simulink model "pv_model"  (R2020a)
settings: Solver=VariableStepAuto  StartTime=0.0  StopTime=10  RelTol=1e-3
undefined symbols (not defined in the file): Eg0, Isc, K, Ki, n, Ns, q, Rs, Rsh, sigbuilder_block, Tn, Voc
libraries: powerlib x12, simulink x11, re_lib x1
settings Model: Creator=vardh  LastModifiedBy=sameeraa
settings SolverCC: AlgebraicLoopSolver=LineSearch
settings DebuggingCC: AlgebraicLoopMsg=none

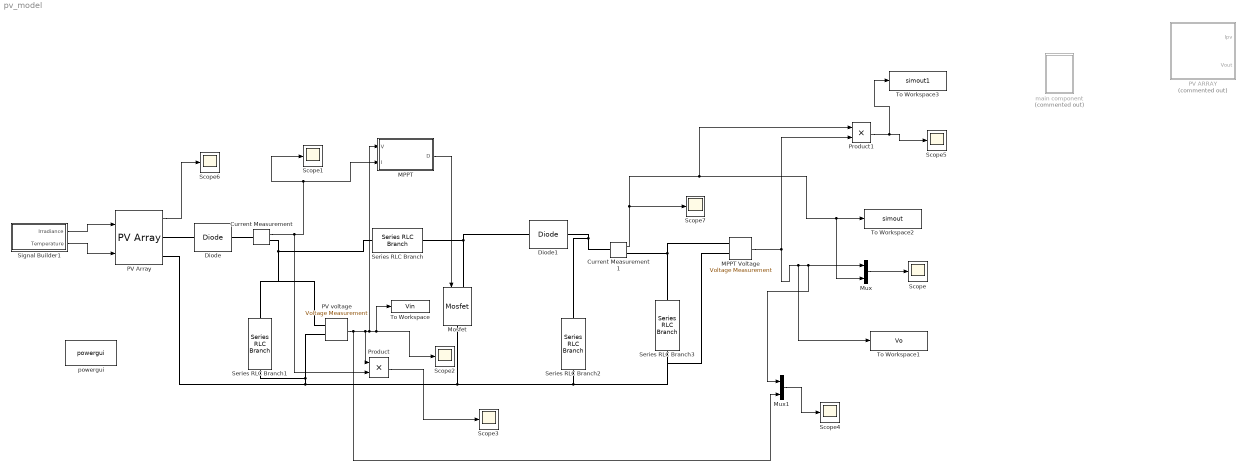
== system pv_model ==
  Current Measurement : powerlib/Measurements/Current Measurement  PhasorSimulation=off  OutputType=Complex  PSBequivalent=0
  Current Measurement1 : powerlib/Measurements/Current Measurement  PhasorSimulation=off  OutputType=Complex  PSBequivalent=0
  Diode : powerlib/Power Electronics/Diode  Ron=0.001  Lon=0  Vf=0.8  IC=0  UseSnubber=0  Rs=500  Cs=250e-9  Measurements=off
  Diode1 : powerlib/Power Electronics/Diode  Ron=0.001  Lon=0  Vf=0.8  IC=0  UseSnubber=0  Rs=500  Cs=250e-9  Measurements=off
  MPPT : Subsystem
  MPPT Voltage : powerlib/Measurements/Voltage Measurement  PhasorSimulation=off  OutputType=Complex  PSBequivalent=0
  Mosfet : powerlib/Power Electronics/Mosfet  Ron=0.1  Lon=0  Rd=0.01  Vfd=0  IC=0  Rs=1e5  Cs=inf  Measurements=off
  Mux : Mux  Inputs=2
  Mux1 : Mux  Inputs=2
  PV ARRAY : Subsystem  Commented=on
  PV Array : re_lib/Solar/PV Array  Npar=1  Nser=1  PlotType=one module @ 25 deg.C & specified irradiances  S_vec="[ 1000  800  600 ]"  Temp_C_vec="[ 45 25  ]"  ModuleName=User-defined  PlotWhenSelected=off  Pm=223.3  Ncell=60  Voc=36.3  Isc=7.84  Vm=29  Im=7.7  beta_Voc_pc=-0.36099  alpha_Isc_pc=0.102  beta_Voc=-0.13104  alpha_Isc=0.0079968  IL=8.0515  I0=2.9406e-10  nI=0.97985  Rsh=6175.6519  Rs=0.38059  RobustModel=off  RobustCellTemperature=25  BAL=on  Tc=1e-6  Tfilter=5e-5
  PV voltage : powerlib/Measurements/Voltage Measurement  PhasorSimulation=off  OutputType=Complex  PSBequivalent=0
  Product : Product
  Product1 : Product
  Scope{,1..7} (8 alike) : Scope
  Series RLC Branch : powerlib/Elements/Series RLC Branch  LConnTagsString=__new0  RConnTagsString=__new0  BranchType=L  Resistance=1  Inductance=1e-3  SetiL0=off  InitialCurrent=0  Capacitance=1e-6  Setx0=off  InitialVoltage=0  Measurements=None
  Series RLC Branch1 : powerlib/Elements/Series RLC Branch  LConnTagsString=__new0  RConnTagsString=__new0  BranchType=C  Resistance=1  Inductance=1e-3  SetiL0=off  InitialCurrent=0  Capacitance=1e-6  Setx0=off  InitialVoltage=0  Measurements=None
  Series RLC Branch2 : powerlib/Elements/Series RLC Branch  LConnTagsString=__new0  RConnTagsString=__new0  BranchType=C  Resistance=1  Inductance=1e-3  SetiL0=off  InitialCurrent=0  Capacitance=1e-6  Setx0=off  InitialVoltage=0  Measurements=None
  Series RLC Branch3 : powerlib/Elements/Series RLC Branch  LConnTagsString=__new0  RConnTagsString=__new0  BranchType=R  Resistance=1  Inductance=1e-3  SetiL0=off  InitialCurrent=0  Capacitance=1e-6  Setx0=off  InitialVoltage=0  Measurements=None
  Signal Builder1 : Subsystem  Tag=STV Subsys  LoadFcn=sigbuilder_block('load');  StartFcn=sigbuilder_block('start');  StopFcn=sigbuilder_block('stop');  ClipboardFcn=sigbuilder_block('clipboard');  mask(Sigbuilder block){tuvar=[0:10]}
      mask help: Simulink:masks:SigbuilderBlock_MD
      mask init:
      | if ~strcmp(get_param(bdroot(gcbh),'SimulationStatus'),'stopped') tuvar = sigbuilder_block('maskInit'); end
      settings: CopyFcn=sigbuilder_block('copy');  DeleteFcn=sigbuilder_block('delete');  ModelCloseFcn=sigbuilder_block('modelClose');  PreSaveFcn=sigbuilder_block('preSave');  PauseFcn=sigbuilder_block('pause');  ContinueFcn=sigbuilder_block('continue');  NameChangeFcn=sigbuilder_block('namechange');  OpenFcn=sigbuilder_block('open',[382.8 123 550.8 400.2 ]);  CloseFcn=sigbuilder_block('close');
      mask Display: plot(0, 0, 100, 100,[2, 2, 32, 32, 2], [68, 8, 8, 68, 68],[32, 2], [38, 38], [32, 19, 2],[53, 60, 44], [32, 17, 17, 2],[16, 16, 31, 31]);txt = getActiveGroup(gcbh);text(2, 100, txt,'verticalAlignment', 'top');
  To Workspace : ToWorkspace  VariableName=Vin  SampleTime=-1
  To Workspace1 : ToWorkspace  VariableName=Vo  SampleTime=-1
  To Workspace2 : ToWorkspace  VariableName=simout  SaveFormat=Timeseries  SampleTime=-1
  To Workspace3 : ToWorkspace  VariableName=simout1  SaveFormat=Timeseries  SampleTime=-1
  main component : Subsystem  Commented=on
  powergui : powerlib/powergui  Priority=1  SimulationMode=Continuous  SampleTime=50e-6  frequency=60  Iterations=50  frequencyindice=0  Pbase=100e6  ErrMax=1e-4  UnitsV=kV  UnitsW=MW  buscounter=0  FunctionMessages=off  echomessages=off  EnableUseOfTLC=off  CurrentSourceSwitches=off  DisableSnubberDevices=off  DisableRonSwitches=off  DisableVfSwitches=off  DisplayEquations=off  AutomaticDiscreteSolvers=off  SolverType=Tustin/Backward Euler (TBE)  Interpol=off  ExternalGateDelay=off  methode=off  Ts=100  x0status=blocks  SPID=on  SwTol=0  HookPort=off  NonlinearTolerance=1e-4  nMaxIteration=100  ContinueOnMaxIteration=off  RestoreLinks=warning  ResistiveCurrentMeasurement=off  Frange=[0:2:500]  Ylog=off  Xlog=on  ShowGrid=off  save=off  variable=ZData  structure=0  ZoomFFT=off  StartTime=0.0  cycles=1  DisplayStyle=1  fundamental=60  FreqAxis=off  MaxFrequency=1000  frequencyindicesteady=1  RmsSteady=1  display=off
  wires:
  Signal Builder1/1(Irradiance) -> PV Array/1
  Signal Builder1/2(Temperature) -> PV Array/2
  Current Measurement/1 -> Product/2, Scope1/1, MPPT/2(I)
  MPPT/1(D) -> Mosfet/1
  PV voltage/1 -> Scope2/1, To Workspace/1, MPPT/1(V), Product/1, Mux1/2
  Product/1 -> Scope3/1
  MPPT Voltage/1 -> To Workspace1/1, Mux/1, Mux1/1, Product1/2
  Mux/1 -> Scope/1
  Mux1/1 -> Scope4/1
  Current Measurement1/1 -> Scope7/1, Product1/1, To Workspace2/1, Mux/2
  Product1/1 -> To Workspace3/1, Scope5/1
  PV Array/1 -> Scope6/1
  connections:
  Diode/RConn1 -- Current Measurement/LConn1
  PV Array/RConn1 -- Diode/LConn1
  Series RLC Branch/LConn1 -- Current Measurement/RConn1 -- PV voltage/LConn1 -- Series RLC Branch1/LConn1
  Series RLC Branch/RConn1 -- Diode1/LConn1 -- Mosfet/LConn1
  Diode1/RConn1 -- Series RLC Branch2/LConn1 -- Current Measurement1/LConn1
  PV Array/RConn2 -- MPPT Voltage/LConn2 -- Series RLC Branch3/RConn1 -- Series RLC Branch2/RConn1 -- Mosfet/RConn1 -- PV voltage/LConn2 -- Series RLC Branch1/RConn1
  Current Measurement1/RConn1 -- Series RLC Branch3/LConn1 -- MPPT Voltage/LConn1

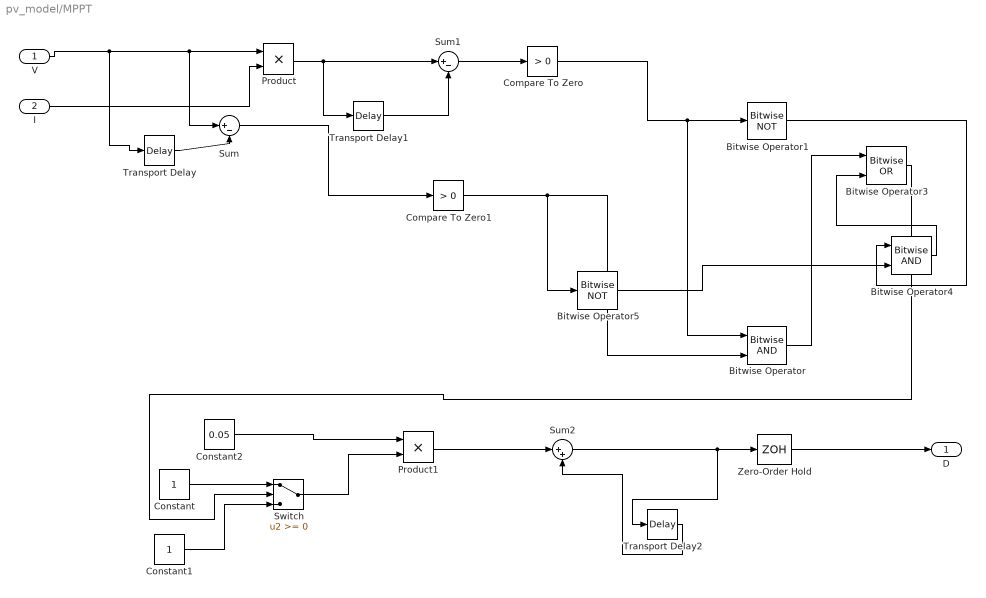
== system pv_model/MPPT ==
  V : Inport
  I : Inport  Port=2
  Bitwise Operator : simulink/Logic and Bit Operations/Bitwise Operator  logicop=AND  UseBitMask=off  NumInputPorts=2  BitMask=bin2dec('11011001')  BitMaskRealWorld=Real World Value
  Bitwise Operator1 : simulink/Logic and Bit Operations/Bitwise Operator  logicop=NOT  UseBitMask=off  BitMask=bin2dec('11011001')  BitMaskRealWorld=Real World Value
  Bitwise Operator3 : simulink/Logic and Bit Operations/Bitwise Operator  logicop=OR  UseBitMask=off  NumInputPorts=2  BitMask=bin2dec('11011001')  BitMaskRealWorld=Real World Value
  Bitwise Operator4 : simulink/Logic and Bit Operations/Bitwise Operator  logicop=AND  UseBitMask=off  NumInputPorts=2  BitMask=bin2dec('11011001')  BitMaskRealWorld=Real World Value
  Bitwise Operator5 : simulink/Logic and Bit Operations/Bitwise Operator  logicop=NOT  UseBitMask=off  BitMask=bin2dec('11011001')  BitMaskRealWorld=Real World Value
  Compare To Zero : simulink/Logic and Bit Operations/Compare To Zero  relop=>  OutDataTypeStr=uint8
  Compare To Zero1 : simulink/Logic and Bit Operations/Compare To Zero  relop=>  OutDataTypeStr=uint8
  Constant : Constant
  Constant1 : Constant
  Constant2 : Constant  Value=0.05
  Product : Product  RndMeth=Zero
  Product1 : Product  RndMeth=Zero
  Sum : Sum  Inputs=|+-
  Sum1 : Sum  Inputs=|+-
  Sum2 : Sum  Inputs=|++
  Switch : Switch
  Transport Delay : TransportDelay  BufferSize=5120
  Transport Delay1 : TransportDelay  DelayTime=10  BufferSize=11264
  Transport Delay2 : TransportDelay  BufferSize=5120
  Zero-Order Hold : ZeroOrderHold
  D : Outport
  wires:
  V/1 -> Product/1, Sum/1, Transport Delay/1
  Transport Delay/1 -> Sum/2
  I/1 -> Product/2
  Product/1 -> Sum1/1, Transport Delay1/1
  Transport Delay1/1 -> Sum1/2
  Sum1/1 -> Compare To Zero/1
  Compare To Zero/1 -> Bitwise Operator1/1, Bitwise Operator/1
  Bitwise Operator/1 -> Bitwise Operator3/1
  Sum/1 -> Compare To Zero1/1
  Compare To Zero1/1 -> Bitwise Operator/2, Bitwise Operator5/1
  Bitwise Operator1/1 -> Bitwise Operator4/1
  Bitwise Operator4/1 -> Bitwise Operator3/2
  Bitwise Operator5/1 -> Bitwise Operator4/2
  Constant/1 -> Switch/1
  Constant1/1 -> Switch/3
  Bitwise Operator3/1 -> Switch/2
  Constant2/1 -> Product1/1
  Switch/1 -> Product1/2
  Product1/1 -> Sum2/1
  Sum2/1 -> Zero-Order Hold/1, Transport Delay2/1
  Transport Delay2/1 -> Sum2/2
  Zero-Order Hold/1 -> D/1

== system pv_model/PV ARRAY ==
  PV Module1 : Subsystem  InitFcn=|
      | Ki=0.0032;
      | q=1.6e-19;
      | K=1.38e-23;
      | n=1.3;
      | Eg0=1.1;
      | Rs=0.221;
      | Rsh=415.405;
      | Tn=298;
      | Voc=32.9;
      | Isc=8.21;
      | Ns=54;
  Ramp2 : simulink/Sources/Ramp  slope=10  start=0  InitialOutput=0
  Signal Builder1 : Subsystem  Tag=STV Subsys  LoadFcn=sigbuilder_block('load');  StartFcn=sigbuilder_block('start');  StopFcn=sigbuilder_block('stop');  ClipboardFcn=sigbuilder_block('clipboard');  mask(Sigbuilder block){tuvar=[0:10]}
      mask help: Simulink:masks:SigbuilderBlock_MD
      mask init:
      | if ~strcmp(get_param(bdroot(gcbh),'SimulationStatus'),'stopped') tuvar = sigbuilder_block('maskInit'); end
      settings: CopyFcn=sigbuilder_block('copy');  DeleteFcn=sigbuilder_block('delete');  ModelCloseFcn=sigbuilder_block('modelClose');  PreSaveFcn=sigbuilder_block('preSave');  PauseFcn=sigbuilder_block('pause');  ContinueFcn=sigbuilder_block('continue');  NameChangeFcn=sigbuilder_block('namechange');  OpenFcn=sigbuilder_block('open',[382.8 123 550.8 400.2 ]);  CloseFcn=sigbuilder_block('close');
      mask Display: plot(0, 0, 100, 100,[2, 2, 32, 32, 2], [68, 8, 8, 68, 68],[32, 2], [38, 38], [32, 19, 2],[53, 60, 44], [32, 17, 17, 2],[16, 16, 31, 31]);txt = getActiveGroup(gcbh);text(2, 100, txt,'verticalAlignment', 'top');
  Ipv : Outport
  Vout : Outport  Port=2
  wires:
  Ramp2/1 -> PV Module1/3(Vin)
  Signal Builder1/2(Temperature) -> PV Module1/1(Temperature)
  PV Module1/2(Vout) -> Vout/1
  Signal Builder1/1(Irradiance) -> PV Module1/2(Irradiance)
  PV Module1/1(Ipv) -> Ipv/1

== system pv_model/Signal Builder1 ==
  Demux : Demux  Tag=STV Demux  Outputs=2
      settings: DisplayOption=none
  FromWs : FromWorkspace  Tag=STV FromWs  VariableName=tuvar
      SigBuilderData=|
      | common.afterFinalStr = 'Extrapolate'
      | common.sampleTime = 0
      | dataSet.timeRange = [0 10]
      | dataSet.name = 'Group 1'
      | sbobj.Groups.Name = 'Group 1'
      | sbobj.Groups.Signals(1).Name = 'Irradiance'
      | sbobj.Groups.Signals(1).XData = [0 10]
      | sbobj.Groups.Signals(1).YData = [1000 1000]
      | sbobj.Groups.Signals(2).Name = 'Temperature'
      | sbobj.Groups.Signals(2).XData = [0 10]
      | sbobj.Groups.Signals(2).YData = [25 25]
  Irradiance : Outport  Tag=STV Outport
  Temperature : Outport  Tag=STV Outport  Port=2
  wires:
  Demux/1 -> Irradiance/1
  FromWs/1 -> Demux/1
  Demux/2 -> Temperature/1

== system pv_model/main component ==
  I-V 1 : simulink/Sinks/XY Graph  xmin=0  xmax=35  ymin=0  ymax=10  st=-1
  P-V1 : simulink/Sinks/XY Graph  xmin=0  xmax=35  ymin=0  ymax=210  st=-1
  PV Module1 : Subsystem  InitFcn=|
      | Ki=0.0032;
      | q=1.6e-19;
      | K=1.38e-23;
      | n=1.3;
      | Eg0=1.1;
      | Rs=0.221;
      | Rsh=415.405;
      | Tn=298;
      | Voc=32.9;
      | Isc=8.21;
      | Ns=54;
  Product1 : Product
  Ramp2 : simulink/Sources/Ramp  slope=10  start=0  InitialOutput=0
  Scope{,1..3} (4 alike) : Scope
  Signal Builder1 : Subsystem  Tag=STV Subsys  LoadFcn=sigbuilder_block('load');  StartFcn=sigbuilder_block('start');  StopFcn=sigbuilder_block('stop');  ClipboardFcn=sigbuilder_block('clipboard');  mask(Sigbuilder block){tuvar=[0:10]}
      mask help: Simulink:masks:SigbuilderBlock_MD
      mask init:
      | if ~strcmp(get_param(bdroot(gcbh),'SimulationStatus'),'stopped') tuvar = sigbuilder_block('maskInit'); end
      settings: CopyFcn=sigbuilder_block('copy');  DeleteFcn=sigbuilder_block('delete');  ModelCloseFcn=sigbuilder_block('modelClose');  PreSaveFcn=sigbuilder_block('preSave');  PauseFcn=sigbuilder_block('pause');  ContinueFcn=sigbuilder_block('continue');  NameChangeFcn=sigbuilder_block('namechange');  OpenFcn=sigbuilder_block('open',[382.8 123 550.8 400.2 ]);  CloseFcn=sigbuilder_block('close');
      mask Display: plot(0, 0, 100, 100,[2, 2, 32, 32, 2], [68, 8, 8, 68, 68],[32, 2], [38, 38], [32, 19, 2],[53, 60, 44], [32, 17, 17, 2],[16, 16, 31, 31]);txt = getActiveGroup(gcbh);text(2, 100, txt,'verticalAlignment', 'top');
  wires:
  PV Module1/2(Vout) -> Scope/1, Product1/2, P-V1/1, I-V 1/1
  Product1/1 -> Scope1/1, P-V1/2
  PV Module1/1(Ipv) -> Scope2/1, Product1/1, I-V 1/2
  Signal Builder1/2(Temperature) -> PV Module1/1(Temperature)
  Ramp2/1 -> Scope3/1, PV Module1/3(Vin)
  Signal Builder1/1(Irradiance) -> PV Module1/2(Irradiance)

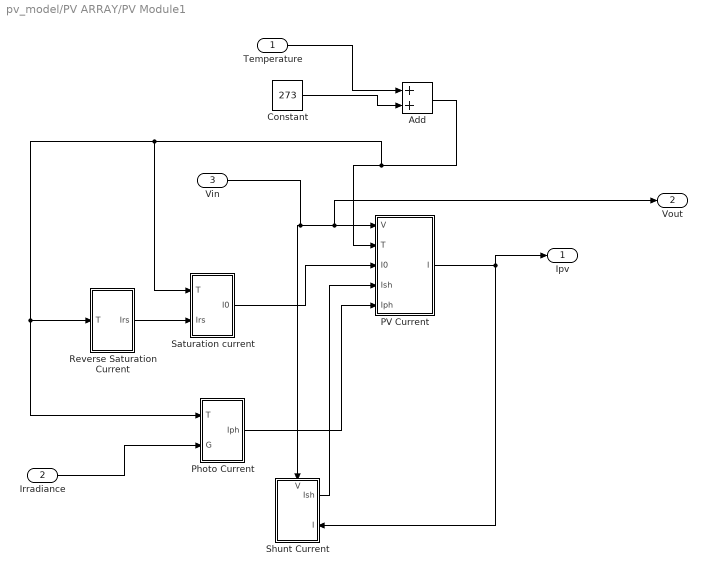
== system pv_model/PV ARRAY/PV Module1 ==
  Temperature : Inport
  Irradiance : Inport  Port=2
  Vin : Inport  Port=3
  Add : Sum
  Constant : Constant  Value=273
  PV Current : Subsystem
  Photo Current : Subsystem
  Reverse Saturation Current : Subsystem
  Saturation current : Subsystem
  Shunt Current : Subsystem
      settings: PortSchema="{\"entries\":[{\"content\":{\"sides\":[{\"content\":{\"connectorIds\":[]},\"type\":\"ConnectorPlacement.EquallySpacedRectSide\",\"uuid\":\"dfbb4c5d-8fcf-4819-9965-5f47220c7753\"},{\"content\":{\"connectorIds\":[\"Out1\",\"In2\"],\"side\":\"RIGHT\"},\"type\":\"ConnectorPlacement.EquallySpacedRectSide\",\"uuid\":\"987aa4c6-8b7c-4032-9cd9-5753be429a4d\"},{\"content\":{\"connectorIds\":[\"In1\"],\"side\":\"TOP\"},\"type\":\"ConnectorPlacement.EquallySpacedRectSide\",\"uuid\":\"a02384b8-48a1-4401-ad36-e6b05eaf9311\"}]},\"type\":\"ConnectorPlacement.EquallySpacedConnector\",\"uuid\":\"4fb9e7c8-c8f8-43f6-a1be-daa0a140ff41\"}],\"packageUris\":[\"http://schema.mathworks.com/mf0/Connector/19700101\"],\"version\":\"1.0\"}"
  Ipv : Outport
  Vout : Outport  Port=2
  wires:
  Vin/1 -> Vout/1, PV Current/1(V), Shunt Current/1(V)
  Irradiance/1 -> Photo Current/2(G)
  Constant/1 -> Add/2
  Add/1 -> Saturation current/1(T), Reverse Saturation Current/1(T), Photo Current/1(T), PV Current/2(T)
  PV Current/1(I) -> Ipv/1, Shunt Current/2(I)
  Saturation current/1(I0) -> PV Current/3(I0)
  Temperature/1 -> Add/1
  Reverse Saturation Current/1(Irs) -> Saturation current/2(Irs)
  Photo Current/1(Iph) -> PV Current/5(Iph)
  Shunt Current/1(Ish) -> PV Current/4(Ish)

== system pv_model/PV ARRAY/Signal Builder1 ==
  Demux : Demux  Tag=STV Demux  Outputs=2
      settings: DisplayOption=none
  FromWs : FromWorkspace  Tag=STV FromWs  VariableName=tuvar
      SigBuilderData=|
      | common.afterFinalStr = 'Extrapolate'
      | common.sampleTime = 0
      | dataSet.timeRange = [0 10]
      | dataSet.name = 'Group 1'
      | sbobj.Groups.Name = 'Group 1'
      | sbobj.Groups.Signals(1).Name = 'Irradiance'
      | sbobj.Groups.Signals(1).XData = [0 10]
      | sbobj.Groups.Signals(1).YData = [1000 1000]
      | sbobj.Groups.Signals(2).Name = 'Temperature'
      | sbobj.Groups.Signals(2).XData = [0 10]
      | sbobj.Groups.Signals(2).YData = [25 25]
  Irradiance : Outport  Tag=STV Outport
  Temperature : Outport  Tag=STV Outport  Port=2
  wires:
  Demux/1 -> Irradiance/1
  FromWs/1 -> Demux/1
  Demux/2 -> Temperature/1

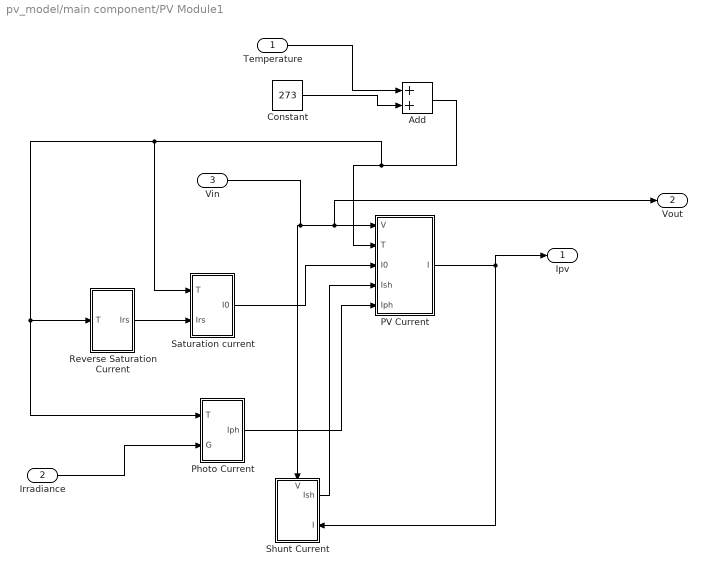
== system pv_model/main component/PV Module1 ==
  Temperature : Inport
  Irradiance : Inport  Port=2
  Vin : Inport  Port=3
  Add : Sum
  Constant : Constant  Value=273
  PV Current : Subsystem
  Photo Current : Subsystem
  Reverse Saturation Current : Subsystem
  Saturation current : Subsystem
  Shunt Current : Subsystem
      settings: PortSchema="{\"entries\":[{\"content\":{\"sides\":[{\"content\":{\"connectorIds\":[]},\"type\":\"ConnectorPlacement.EquallySpacedRectSide\",\"uuid\":\"dfbb4c5d-8fcf-4819-9965-5f47220c7753\"},{\"content\":{\"connectorIds\":[\"Out1\",\"In2\"],\"side\":\"RIGHT\"},\"type\":\"ConnectorPlacement.EquallySpacedRectSide\",\"uuid\":\"987aa4c6-8b7c-4032-9cd9-5753be429a4d\"},{\"content\":{\"connectorIds\":[\"In1\"],\"side\":\"TOP\"},\"type\":\"ConnectorPlacement.EquallySpacedRectSide\",\"uuid\":\"a02384b8-48a1-4401-ad36-e6b05eaf9311\"}]},\"type\":\"ConnectorPlacement.EquallySpacedConnector\",\"uuid\":\"4fb9e7c8-c8f8-43f6-a1be-daa0a140ff41\"}],\"packageUris\":[\"http://schema.mathworks.com/mf0/Connector/19700101\"],\"version\":\"1.0\"}"
  Ipv : Outport
  Vout : Outport  Port=2
  wires:
  Vin/1 -> Vout/1, PV Current/1(V), Shunt Current/1(V)
  Irradiance/1 -> Photo Current/2(G)
  Constant/1 -> Add/2
  Add/1 -> Saturation current/1(T), Reverse Saturation Current/1(T), Photo Current/1(T), PV Current/2(T)
  PV Current/1(I) -> Ipv/1, Shunt Current/2(I)
  Saturation current/1(I0) -> PV Current/3(I0)
  Temperature/1 -> Add/1
  Reverse Saturation Current/1(Irs) -> Saturation current/2(Irs)
  Photo Current/1(Iph) -> PV Current/5(Iph)
  Shunt Current/1(Ish) -> PV Current/4(Ish)

== system pv_model/main component/Signal Builder1 ==
  Demux : Demux  Tag=STV Demux  Outputs=2
      settings: DisplayOption=none
  FromWs : FromWorkspace  Tag=STV FromWs  VariableName=tuvar
      SigBuilderData=|
      | common.afterFinalStr = 'Extrapolate'
      | common.sampleTime = 0
      | dataSet.timeRange = [0 10]
      | dataSet.name = 'Group 1'
      | sbobj.Groups.Name = 'Group 1'
      | sbobj.Groups.Signals(1).Name = 'Irradiance'
      | sbobj.Groups.Signals(1).XData = [0 10]
      | sbobj.Groups.Signals(1).YData = [1000 1000]
      | sbobj.Groups.Signals(2).Name = 'Temperature'
      | sbobj.Groups.Signals(2).XData = [0 10]
      | sbobj.Groups.Signals(2).YData = [25 25]
  Irradiance : Outport  Tag=STV Outport
  Temperature : Outport  Tag=STV Outport  Port=2
  wires:
  Demux/1 -> Irradiance/1
  FromWs/1 -> Demux/1
  Demux/2 -> Temperature/1

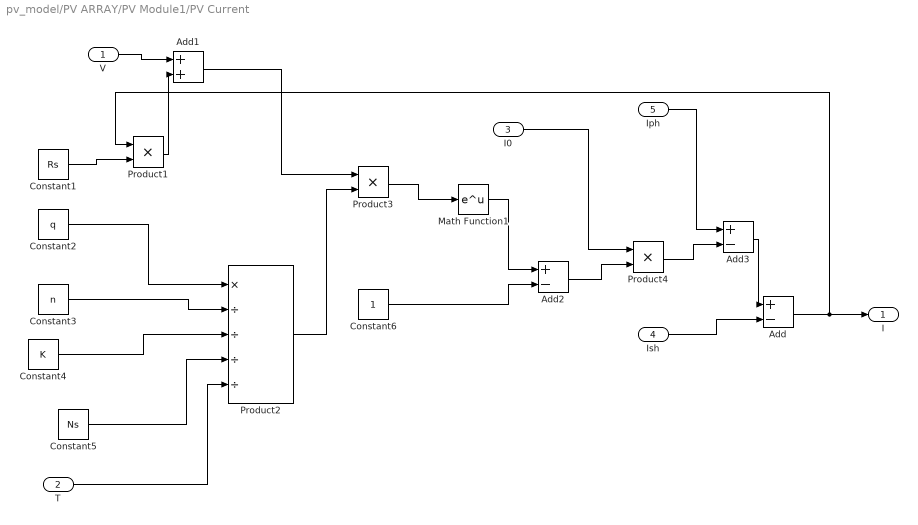
== system pv_model/PV ARRAY/PV Module1/PV Current ==
  V : Inport
  T : Inport  Port=2
  I0 : Inport  Port=3
  Ish : Inport  Port=4
  Iph : Inport  Port=5
  Add : Sum  Inputs=+-
  Add1 : Sum
  Add2 : Sum  Inputs=+-
  Add3 : Sum  Inputs=+-
  Constant1 : Constant  Value=Rs
  Constant2 : Constant  Value=q
  Constant3 : Constant  Value=n
  Constant4 : Constant  Value=K
  Constant5 : Constant  Value=Ns
  Constant6 : Constant
  Math Function1 : Math  SaturateOnIntegerOverflow=on
  Product1 : Product
  Product2 : Product  Inputs=*////
  Product3 : Product
  Product4 : Product
  I : Outport
  wires:
  Product3/1 -> Math Function1/1
  Constant1/1 -> Product1/2
  Add3/1 -> Add/1
  T/1 -> Product2/5
  Constant5/1 -> Product2/4
  Constant2/1 -> Product2/1
  Add2/1 -> Product4/2
  Constant3/1 -> Product2/2
  Constant4/1 -> Product2/3
  Product2/1 -> Product3/2
  Iph/1 -> Add3/1
  Math Function1/1 -> Add2/1
  Product4/1 -> Add3/2
  V/1 -> Add1/1
  Add/1 -> I/1, Product1/1
  Constant6/1 -> Add2/2
  Product1/1 -> Add1/2
  I0/1 -> Product4/1
  Add1/1 -> Product3/1
  Ish/1 -> Add/2

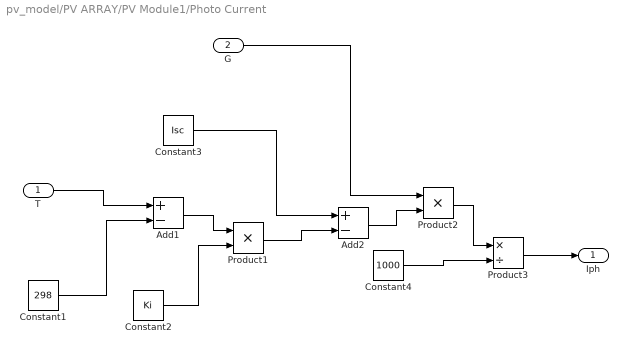
== system pv_model/PV ARRAY/PV Module1/Photo Current ==
  T : Inport
  G : Inport  Port=2
  Add1 : Sum  Inputs=+-
  Add2 : Sum  Inputs=+-
  Constant1 : Constant  Value=298
  Constant2 : Constant  Value=Ki
  Constant3 : Constant  Value=Isc
  Constant4 : Constant  Value=1000
  Product1 : Product
  Product2 : Product
  Product3 : Product  Inputs=*/
  Iph : Outport
  wires:
  Add2/1 -> Product2/2
  Constant3/1 -> Add2/1
  Constant4/1 -> Product3/2
  Product3/1 -> Iph/1
  Product1/1 -> Add2/2
  Add1/1 -> Product1/1
  G/1 -> Product2/1
  Product2/1 -> Product3/1
  Constant1/1 -> Add1/2
  T/1 -> Add1/1
  Constant2/1 -> Product1/2

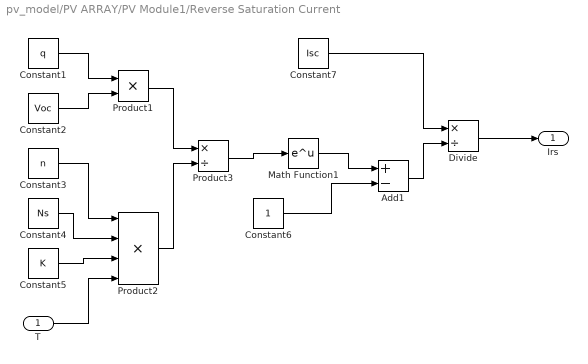
== system pv_model/PV ARRAY/PV Module1/Reverse Saturation Current ==
  T : Inport
  Add1 : Sum  Inputs=+-
  Constant1 : Constant  Value=q
  Constant2 : Constant  Value=Voc
  Constant3 : Constant  Value=n
  Constant4 : Constant  Value=Ns
  Constant5 : Constant  Value=K
  Constant6 : Constant
  Constant7 : Constant  Value=Isc
  Divide : Product  Inputs=*/
  Math Function1 : Math  SaturateOnIntegerOverflow=on
  Product1 : Product
  Product2 : Product  Inputs=4
  Product3 : Product  Inputs=*/
  Irs : Outport
  wires:
  Product2/1 -> Product3/2
  Constant3/1 -> Product2/1
  Constant6/1 -> Add1/2
  Constant4/1 -> Product2/2
  Constant2/1 -> Product1/2
  Product1/1 -> Product3/1
  Constant5/1 -> Product2/3
  Math Function1/1 -> Add1/1
  Constant1/1 -> Product1/1
  Divide/1 -> Irs/1
  Product3/1 -> Math Function1/1
  T/1 -> Product2/4
  Add1/1 -> Divide/2
  Constant7/1 -> Divide/1

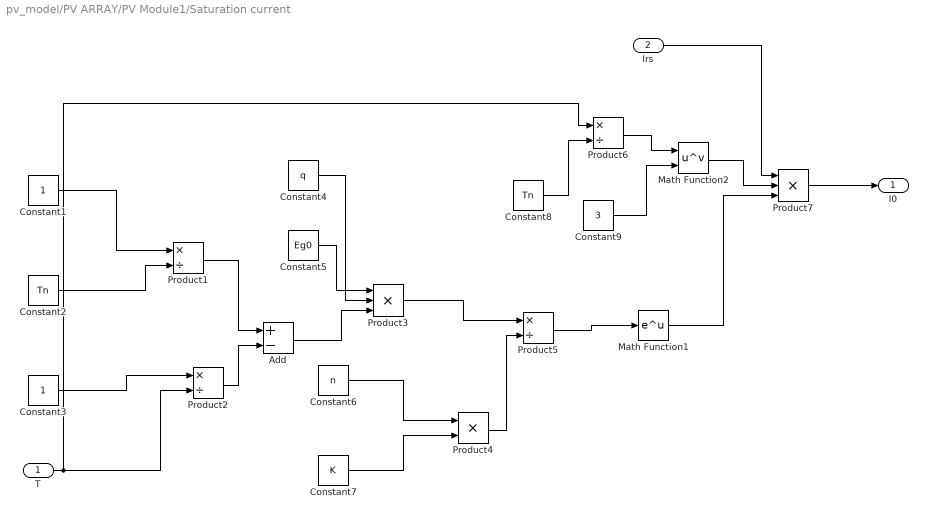
== system pv_model/PV ARRAY/PV Module1/Saturation current ==
  T : Inport
  Irs : Inport  Port=2
  Add : Sum  Inputs=+-
  Constant1 : Constant
  Constant2 : Constant  Value=Tn
  Constant3 : Constant
  Constant4 : Constant  Value=q
  Constant5 : Constant  Value=Eg0
  Constant6 : Constant  Value=n
  Constant7 : Constant  Value=K
  Constant8 : Constant  Value=Tn
  Constant9 : Constant  Value=3
  Math Function1 : Math  SaturateOnIntegerOverflow=on
  Math Function2 : Math  Operator=pow  SaturateOnIntegerOverflow=on
  Product{1..2,5..6} (4 alike) : Product  Inputs=*/
  Product3 : Product  Inputs=***
  Product4 : Product
  Product7 : Product  Inputs=3
  I0 : Outport
  wires:
  Product7/1 -> I0/1
  Constant1/1 -> Product1/1
  Constant2/1 -> Product1/2
  Product4/1 -> Product5/2
  Constant9/1 -> Math Function2/2
  Product3/1 -> Product5/1
  Constant6/1 -> Product4/1
  Add/1 -> Product3/3
  Irs/1 -> Product7/1
  T/1 -> Product2/2, Product6/1
  Math Function2/1 -> Product7/2
  Constant5/1 -> Product3/1
  Math Function1/1 -> Product7/3
  Constant8/1 -> Product6/2
  Product6/1 -> Math Function2/1
  Product1/1 -> Add/1
  Product5/1 -> Math Function1/1
  Constant3/1 -> Product2/1
  Product2/1 -> Add/2
  Constant4/1 -> Product3/2
  Constant7/1 -> Product4/2

== system pv_model/PV ARRAY/PV Module1/Shunt Current ==
  V : Inport
  I : Inport  Port=2
  Add1 : Sum
  Constant1 : Constant  Value=Rs
  Constant2 : Constant  Value=Rsh
  Divide : Product  Inputs=*/
  Product1 : Product
  Ish : Outport
  wires:
  Add1/1 -> Divide/1
  Product1/1 -> Add1/1
  I/1 -> Product1/1
  Constant2/1 -> Divide/2
  Constant1/1 -> Product1/2
  Divide/1 -> Ish/1
  V/1 -> Add1/2

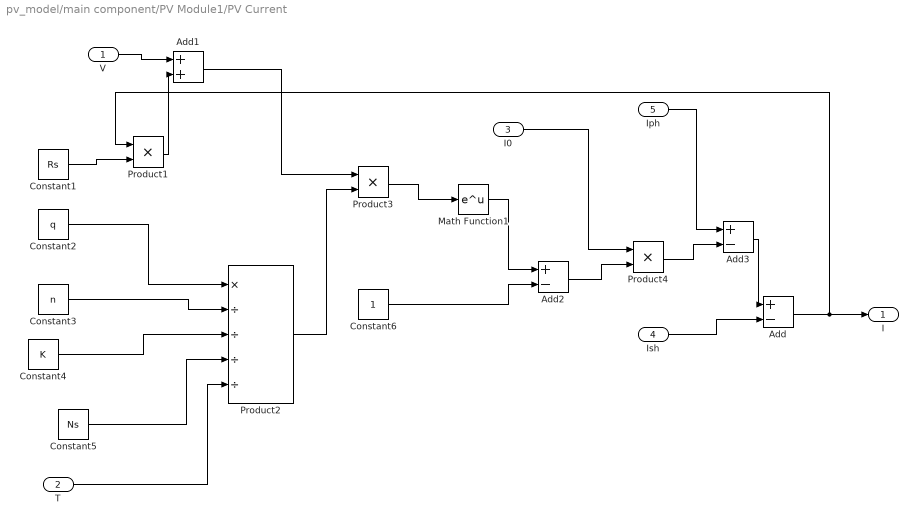
== system pv_model/main component/PV Module1/PV Current ==
  V : Inport
  T : Inport  Port=2
  I0 : Inport  Port=3
  Ish : Inport  Port=4
  Iph : Inport  Port=5
  Add : Sum  Inputs=+-
  Add1 : Sum
  Add2 : Sum  Inputs=+-
  Add3 : Sum  Inputs=+-
  Constant1 : Constant  Value=Rs
  Constant2 : Constant  Value=q
  Constant3 : Constant  Value=n
  Constant4 : Constant  Value=K
  Constant5 : Constant  Value=Ns
  Constant6 : Constant
  Math Function1 : Math  SaturateOnIntegerOverflow=on
  Product1 : Product
  Product2 : Product  Inputs=*////
  Product3 : Product
  Product4 : Product
  I : Outport
  wires:
  Product3/1 -> Math Function1/1
  Constant1/1 -> Product1/2
  Add3/1 -> Add/1
  T/1 -> Product2/5
  Constant5/1 -> Product2/4
  Constant2/1 -> Product2/1
  Add2/1 -> Product4/2
  Constant3/1 -> Product2/2
  Constant4/1 -> Product2/3
  Product2/1 -> Product3/2
  Iph/1 -> Add3/1
  Math Function1/1 -> Add2/1
  Product4/1 -> Add3/2
  V/1 -> Add1/1
  Add/1 -> I/1, Product1/1
  Constant6/1 -> Add2/2
  Product1/1 -> Add1/2
  I0/1 -> Product4/1
  Add1/1 -> Product3/1
  Ish/1 -> Add/2

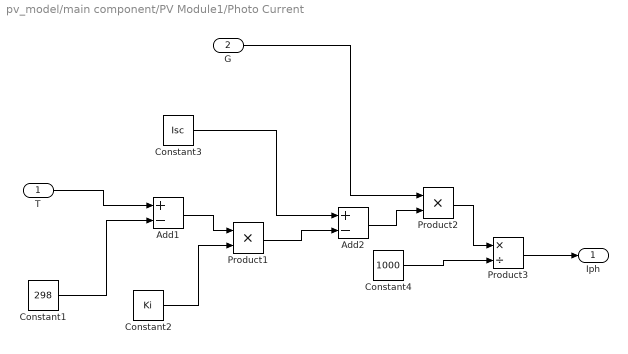
== system pv_model/main component/PV Module1/Photo Current ==
  T : Inport
  G : Inport  Port=2
  Add1 : Sum  Inputs=+-
  Add2 : Sum  Inputs=+-
  Constant1 : Constant  Value=298
  Constant2 : Constant  Value=Ki
  Constant3 : Constant  Value=Isc
  Constant4 : Constant  Value=1000
  Product1 : Product
  Product2 : Product
  Product3 : Product  Inputs=*/
  Iph : Outport
  wires:
  Add2/1 -> Product2/2
  Constant3/1 -> Add2/1
  Constant4/1 -> Product3/2
  Product3/1 -> Iph/1
  Product1/1 -> Add2/2
  Add1/1 -> Product1/1
  G/1 -> Product2/1
  Product2/1 -> Product3/1
  Constant1/1 -> Add1/2
  T/1 -> Add1/1
  Constant2/1 -> Product1/2

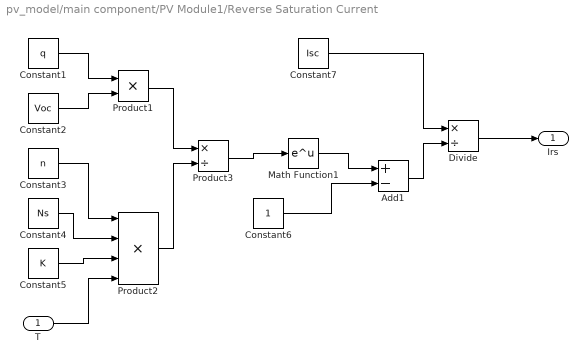
== system pv_model/main component/PV Module1/Reverse Saturation Current ==
  T : Inport
  Add1 : Sum  Inputs=+-
  Constant1 : Constant  Value=q
  Constant2 : Constant  Value=Voc
  Constant3 : Constant  Value=n
  Constant4 : Constant  Value=Ns
  Constant5 : Constant  Value=K
  Constant6 : Constant
  Constant7 : Constant  Value=Isc
  Divide : Product  Inputs=*/
  Math Function1 : Math  SaturateOnIntegerOverflow=on
  Product1 : Product
  Product2 : Product  Inputs=4
  Product3 : Product  Inputs=*/
  Irs : Outport
  wires:
  Product2/1 -> Product3/2
  Constant3/1 -> Product2/1
  Constant6/1 -> Add1/2
  Constant4/1 -> Product2/2
  Constant2/1 -> Product1/2
  Product1/1 -> Product3/1
  Constant5/1 -> Product2/3
  Math Function1/1 -> Add1/1
  Constant1/1 -> Product1/1
  Divide/1 -> Irs/1
  Product3/1 -> Math Function1/1
  T/1 -> Product2/4
  Add1/1 -> Divide/2
  Constant7/1 -> Divide/1

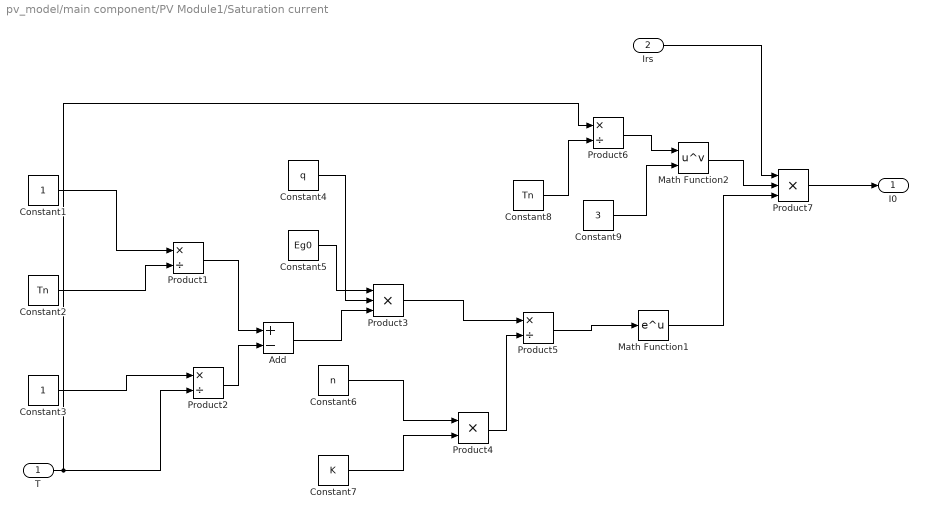
== system pv_model/main component/PV Module1/Saturation current ==
  T : Inport
  Irs : Inport  Port=2
  Add : Sum  Inputs=+-
  Constant1 : Constant
  Constant2 : Constant  Value=Tn
  Constant3 : Constant
  Constant4 : Constant  Value=q
  Constant5 : Constant  Value=Eg0
  Constant6 : Constant  Value=n
  Constant7 : Constant  Value=K
  Constant8 : Constant  Value=Tn
  Constant9 : Constant  Value=3
  Math Function1 : Math  SaturateOnIntegerOverflow=on
  Math Function2 : Math  Operator=pow  SaturateOnIntegerOverflow=on
  Product{1..2,5..6} (4 alike) : Product  Inputs=*/
  Product3 : Product  Inputs=***
  Product4 : Product
  Product7 : Product  Inputs=3
  I0 : Outport
  wires:
  Product7/1 -> I0/1
  Constant1/1 -> Product1/1
  Constant2/1 -> Product1/2
  Product4/1 -> Product5/2
  Constant9/1 -> Math Function2/2
  Product3/1 -> Product5/1
  Constant6/1 -> Product4/1
  Add/1 -> Product3/3
  Irs/1 -> Product7/1
  T/1 -> Product2/2, Product6/1
  Math Function2/1 -> Product7/2
  Constant5/1 -> Product3/1
  Math Function1/1 -> Product7/3
  Constant8/1 -> Product6/2
  Product6/1 -> Math Function2/1
  Product1/1 -> Add/1
  Product5/1 -> Math Function1/1
  Constant3/1 -> Product2/1
  Product2/1 -> Add/2
  Constant4/1 -> Product3/2
  Constant7/1 -> Product4/2

== system pv_model/main component/PV Module1/Shunt Current ==
  V : Inport
  I : Inport  Port=2
  Add1 : Sum
  Constant1 : Constant  Value=Rs
  Constant2 : Constant  Value=Rsh
  Divide : Product  Inputs=*/
  Product1 : Product
  Ish : Outport
  wires:
  Add1/1 -> Divide/1
  Product1/1 -> Add1/1
  I/1 -> Product1/1
  Constant2/1 -> Divide/2
  Constant1/1 -> Product1/2
  Divide/1 -> Ish/1
  V/1 -> Add1/2
